simulink model "Sue_CalibTrainTrike_Constant_Load_NoStim"  (Simulink 6.6)
settings: Solver=FixedStepDiscrete  StartTime=0.0  StopTime=inf  FixedStep=parameters.model.sample_time  RelTol=1e-3
StopFcn:
  |     % Name .mat file
  | 
  |     datime = datestr(now);
  |     colon = datime == ':';
  |     space = datime == ' ';
  |     dash  = datime == '-';
  |     datime(colon) = '';
  |     datime(space) = '_';
  |     datime(dash) = '';
  | 
  |     prompt = {'Subject #?','When? (PRE,POST,etc.)','Type of test? (CONST,WIN,etc)', 'Loaded? (Enter loaded or unloaded)'};
  | 
  |     dlgTitle = 'File Name';
  |     numlines = 1;
  | 
  |     default = {'000','PREPOST','CONSTWIN','loadedunloaded'};
  |     userinfo = inputdlg(prompt,dlgTitle,numlines,default);
  | 
  |     if isempty(userinfo) == 0
  |         sub = userinfo{1};
  |         reltime = userinfo{2};
  |         testype = userinfo{3};
  |         resist  = userinfo{4};
  | 
  |         Filename = strcat('FESCycling_',sub,'_',reltime,'_',testype,'_',resist,'_',datime)
  | 
  | %     cd path_file
  | %
  |         save(Filename)
  |     end
values from neighbouring files (symbols this model uses):
  cad_ref = 30    [FESCycling_30_PRE_CONST_loaded_12Aug2014_085817.mat]    (also in constant_load_load.m = str2double(get(bla,'String')); constant_load_load_Orig.m = str2double(get(bla,'String')); param.m; param_orig.m = 0)
  freq_range = 1022.16    [FESCycling_30_PRE_CONST_loaded_12Aug2014_085817.mat]    (also in constant_load_load.m; constant_load_load_Orig.m = 466.8; param.m; param_orig.m = 865.41)
  freq_zero = -38.15    [FESCycling_30_PRE_CONST_loaded_12Aug2014_085817.mat]    (also in constant_load_load.m; constant_load_load_Orig.m = 116.7756; param.m; param_orig.m = 39.49)
  parameters =     [FESCycling_30_PRE_CONST_loaded_12Aug2014_085817.mat]
  phio_mat = [1 -0.559 0.0775]    [FESCycling_30_PRE_CONST_loaded_12Aug2014_085817.mat]    (also in constant_load_load.m; constant_load_load_Orig.m; param.m; param_orig.m)
  Pstep = 5    [FESCycling_30_PRE_CONST_loaded_12Aug2014_085817.mat]    (also in constant_load_load.m = str2double(get(bla,'String')); constant_load_load_Orig.m = str2double(get(bla,'String')); param.m = 32; param_orig.m = 114)
  Pw = 0    [FESCycling_30_PRE_CONST_loaded_12Aug2014_085817.mat]    (also in constant_load_load.m = str2double(get(bla,'String')); constant_load_load_Orig.m = str2double(get(bla,'String')); param.m; param_orig.m)
  ro_mat = [0.7602 -0.2976 0.0591]    [FESCycling_30_PRE_CONST_loaded_12Aug2014_085817.mat]    (also in constant_load_load.m; constant_load_load_Orig.m; param.m; param_orig.m)
  s_mat = [0.0005025 -0.0003467]    [FESCycling_30_PRE_CONST_loaded_12Aug2014_085817.mat]    (also in constant_load_load.m = [0.5025 -0.3467]*1e-3; constant_load_load_Orig.m = [0.5025 -0.3467]*1e-3; param.m = [0.5025 -0.3467]*1e-3; param_orig.m = [0.5025 -0.3467]*1e-3)
  slope = 15.81    [FESCycling_30_PRE_CONST_loaded_12Aug2014_085817.mat]    (also in constant_load_load.m; constant_load_load_Orig.m = 14.1374; param.m; param_orig.m = 14.1374)
  stim_max = 0.1    [FESCycling_30_PRE_CONST_loaded_12Aug2014_085817.mat]    (also in constant_load_load.m; constant_load_load_Orig.m; param.m = 500; param_orig.m = 0)
  stim_min = 0    [FESCycling_30_PRE_CONST_loaded_12Aug2014_085817.mat]    (also in constant_load_load.m; constant_load_load_Orig.m; param.m; param_orig.m)
  t_mat = [0.0002987 -0.000166 2.31e-05]    [FESCycling_30_PRE_CONST_loaded_12Aug2014_085817.mat]    (also in constant_load_load.m = [0.2987 -0.1660 0.0231]*1e-3; constant_load_load_Orig.m = [0.2987 -0.1660 0.0231]*1e-3; param.m = [0.2987 -0.1660 0.0231]*1e-3; param_orig.m = [0.2987 -0.1660 0.0231]*1e-3)
  Ts = 20    [FESCycling_30_PRE_CONST_loaded_12Aug2014_085817.mat]    (also in constant_load_load.m; constant_load_load_Orig.m; param.m; param_orig.m)
  Tw = 6000    [FESCycling_30_PRE_CONST_loaded_12Aug2014_085817.mat]    (also in constant_load_load.m; constant_load_load_Orig.m; param.m; param_orig.m)
undefined symbols (not defined in the file or in its folder): ansim
libraries: ni_lib x2, Stimulation_Currents_lib x1, stimulation_staticAngles_lib x1
(part 2 of 2)

== system Sue_CalibTrainTrike_Constant_Load_NoStim/Stimulation_System/Serial_Stimulation_System/Stimulation Activation/Angle Check1/0 < start < 360 ==
  In1 : Inport
  Gain : Gain  Gain=360  SaturateOnIntegerOverflow=on
  Gain1 : Gain  Gain=1/360  SaturateOnIntegerOverflow=on
  Rounding Function : Rounding
  Sum : Sum  Inputs=|+-  SaturateOnIntegerOverflow=on  InputSameDT=on
  Out1 : Outport
  wires:
  In1/1 -> Sum/1, Gain1/1
  Gain1/1 -> Rounding Function/1
  Rounding Function/1 -> Gain/1
  Gain/1 -> Sum/2
  Sum/1 -> Out1/1

== system Sue_CalibTrainTrike_Constant_Load_NoStim/Stimulation_System/Serial_Stimulation_System/Stimulation Activation/Angle Check1/0 < stop < 360 ==
  In1 : Inport
  Gain : Gain  Gain=360  SaturateOnIntegerOverflow=on
  Gain1 : Gain  Gain=1/360  SaturateOnIntegerOverflow=on
  Rounding Function : Rounding
  Sum : Sum  Inputs=|+-  SaturateOnIntegerOverflow=on  InputSameDT=on
  Out1 : Outport
  wires:
  Sum/1 -> Out1/1
  Gain/1 -> Sum/2
  Rounding Function/1 -> Gain/1
  Gain1/1 -> Rounding Function/1
  In1/1 -> Gain1/1, Sum/1
